simulink model "motorsLibrary"  (R2016b)
settings: Solver=VariableStepAuto  StartTime=0.0  StopTime=10.0  RelTol=1e-3
undefined symbols (not defined in the file): LD
settings Model: Creator=sork9  LastModifiedBy=sork9

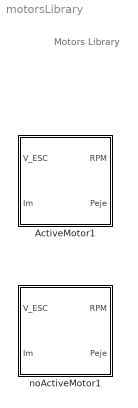
== system motorsLibrary ==
  note: Motors Library
  ActiveMotor1 : Subsystem
  noActiveMotor1 : Subsystem

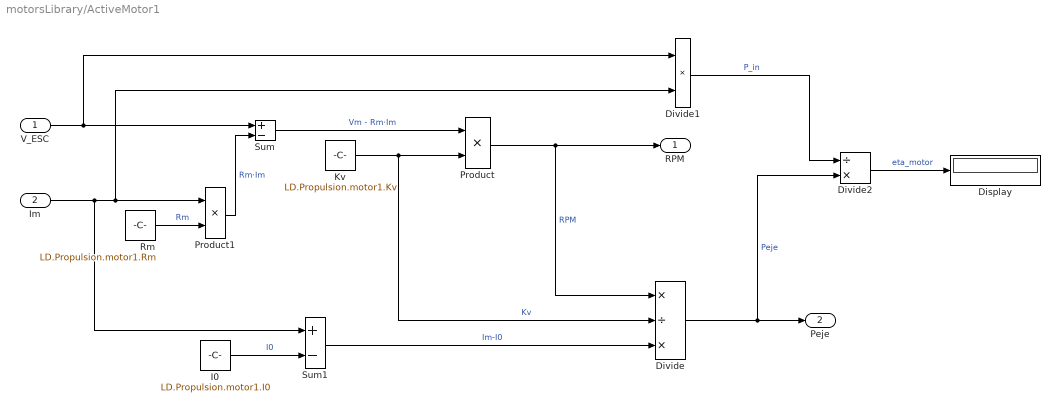
== system motorsLibrary/ActiveMotor1 ==
  V_ESC : Inport
  Im : Inport  Port=2
  Display : Display
  Divide : Product  Inputs=*/*
  Divide1 : Product  Inputs=**
  Divide2 : Product  Inputs=/*
  I0 : Constant  Value=LD.Propulsion.motor1.I0
  Kv : Constant  Value=LD.Propulsion.motor1.Kv
  Product : Product
  Product1 : Product
  Rm : Constant  Value=LD.Propulsion.motor1.Rm
  Sum : Sum  Inputs=+-
  Sum1 : Sum  Inputs=+-
  RPM : Outport
  Peje : Outport  Port=2
  wires:
  I0/1 -> Sum1/2  "I0"
  Divide1/1 -> Divide2/1  "P_in"
  V_ESC/1 -> Divide1/1, Sum/1
  Sum/1 -> Product/1  "Vm - Rm·Im"
  Im/1 -> Sum1/1, Divide1/2, Product1/1
  Divide/1 -> Peje/1, Divide2/2  "Peje"
  Kv/1 -> Divide/2, Product/2  "Kv"
  Product/1 -> RPM/1, Divide/1  "RPM"
  Rm/1 -> Product1/2  "Rm"
  Product1/1 -> Sum/2  "Rm·Im"
  Divide2/1 -> Display/1  "eta_motor"
  Sum1/1 -> Divide/3  "Im-I0"

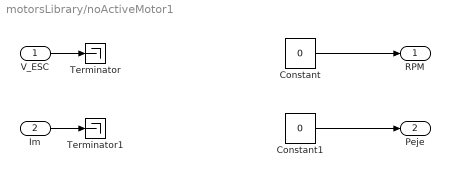
== system motorsLibrary/noActiveMotor1 ==
  V_ESC : Inport
  Im : Inport  Port=2
  Constant : Constant  Value=0
  Constant1 : Constant  Value=0
  Terminator : Terminator
  Terminator1 : Terminator
  RPM : Outport
  Peje : Outport  Port=2
  wires:
  V_ESC/1 -> Terminator/1
  Im/1 -> Terminator1/1
  Constant/1 -> RPM/1
  Constant1/1 -> Peje/1
